simulink model "batteryModel"  (R2024b)
settings: Solver=VariableStepAuto  StartTime=0.0  StopTime=10.0  RelTol=1e-3
model workspace (MAT data in the model file):
  Capacity__Ah_ = 3
  dt = 0.001
undefined symbols (not defined in the file or in its folder): C1_array, Crate_vector, OCV_matrix, R0_array, R1_array, SOC_common, temp_vector
settings Model: Creator=xoxi.1  LastModifiedBy=xoxi.1

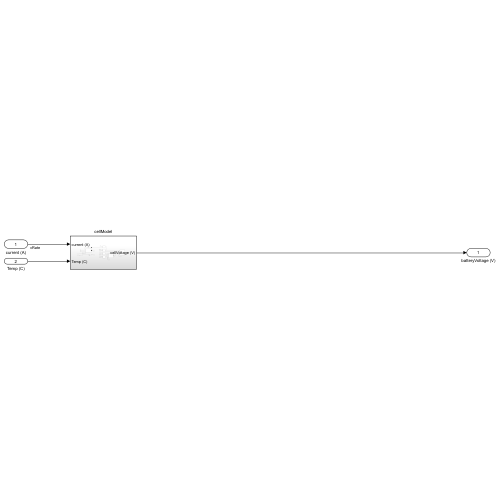
[thumbnail: Simulink's stored preview of the top-level diagram]
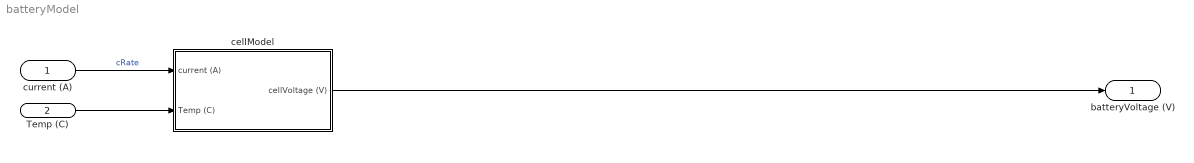
== system batteryModel ==
  current (A) : Inport
  Temp (C) : Inport  Port=2
  cellModel : Subsystem
  batteryVoltage (V) : Outport
  wires:
  current (A)/1 -> cellModel/1(current (A))  "cRate"
  Temp (C)/1 -> cellModel/2(Temp (C))
  cellModel/1(cellVoltage (V)) -> batteryVoltage (V)/1

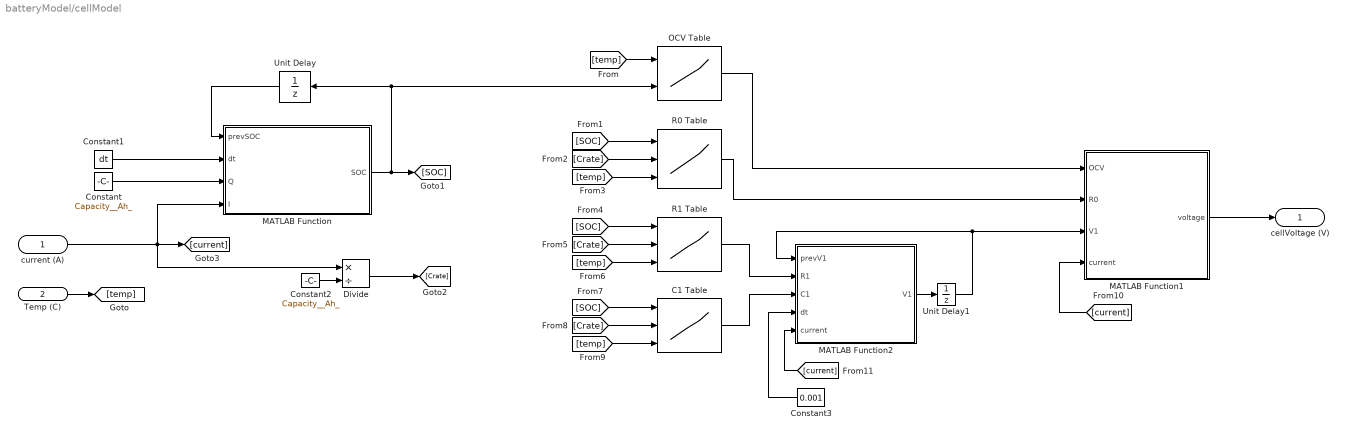
== system batteryModel/cellModel ==
  current (A) : Inport
  Temp (C) : Inport  Port=2
  C1 Table : Lookup_n-D  NumberOfTableDimensions=3  BreakpointsForDimension1=SOC_common  BreakpointsForDimension2=Crate_vector  BreakpointsForDimension3=temp_vector  Table=C1_array  InternalRulePriority=Speed  RndMeth=Simplest
      settings: InputPortMap=u0,u1,u2
  Constant : Constant  Value=Capacity__Ah_
  Constant1 : Constant  Value=dt
  Constant2 : Constant  Value=Capacity__Ah_
  Constant3 : Constant  Value=0.001
  Divide : Product  Inputs=*/
  MATLAB Function : MATLAB Function  TreatAsAtomicUnit=on
  MATLAB Function1 : MATLAB Function  TreatAsAtomicUnit=on
  MATLAB Function2 : MATLAB Function  TreatAsAtomicUnit=on
  OCV Table : Lookup_n-D  BreakpointsForDimension1=temp_vector  BreakpointsForDimension2=SOC_common  Table=OCV_matrix  InternalRulePriority=Speed  RndMeth=Simplest
      settings: InputPortMap=u0,u1
  R0 Table : Lookup_n-D  NumberOfTableDimensions=3  BreakpointsForDimension1=SOC_common  BreakpointsForDimension2=Crate_vector  BreakpointsForDimension3=temp_vector  Table=R0_array  InternalRulePriority=Speed  RndMeth=Simplest
      settings: InputPortMap=u0,u1,u2
  R1 Table : Lookup_n-D  NumberOfTableDimensions=3  BreakpointsForDimension1=SOC_common  BreakpointsForDimension2=Crate_vector  BreakpointsForDimension3=temp_vector  Table=R1_array  InternalRulePriority=Speed  RndMeth=Simplest
      settings: InputPortMap=u0,u1,u2
  Unit Delay : UnitDelay  InitialCondition=1  SampleTime=-1  HasFrameUpgradeWarning=on
  Unit Delay1 : UnitDelay  SampleTime=-1  HasFrameUpgradeWarning=on
  cellVoltage (V) : Outport
  wires:
  R0 Table/1 -> MATLAB Function1/2(R0)
  Unit Delay/1 -> MATLAB Function/1(prevSOC)
  [SOC] -> R0 Table/1
  current (A)/1 -> [current], Divide/1, MATLAB Function/4(I)
  [Crate] -> C1 Table/2
  Constant3/1 -> MATLAB Function2/4(dt)
  Constant1/1 -> MATLAB Function/2(dt)
  [temp] -> C1 Table/3
  [temp] -> R0 Table/3
  [current] -> MATLAB Function2/5(current)
  MATLAB Function1/1(voltage) -> cellVoltage (V)/1
  [temp] -> OCV Table/1
  R1 Table/1 -> MATLAB Function2/2(R1)
  [SOC] -> R1 Table/1
  Constant/1 -> MATLAB Function/3(Q)
  [current] -> MATLAB Function1/4(current)
  Divide/1 -> [Crate]
  Temp (C)/1 -> [temp]
  [SOC] -> C1 Table/1
  MATLAB Function/1(SOC) -> [SOC], Unit Delay/1, OCV Table/2
  MATLAB Function2/1(V1) -> Unit Delay1/1
  [temp] -> R1 Table/3
  Constant2/1 -> Divide/2
  [Crate] -> R0 Table/2
  [Crate] -> R1 Table/2
  OCV Table/1 -> MATLAB Function1/1(OCV)
  Unit Delay1/1 -> MATLAB Function1/3(V1), MATLAB Function2/1(prevV1)
  C1 Table/1 -> MATLAB Function2/3(C1)

== matlab function batteryModel/cellModel/MATLAB Function1 ==
  data: voltage output; OCV input; R0 input; V1 input; current input
function voltage = calculate_voltage(OCV, R0, V1, current)

voltage = OCV - (current * R0) - V1;

end

== matlab function batteryModel/cellModel/MATLAB Function ==
  data: prevSOC input; dt input; Q input; I input; SOC output
function SOC = calculateSOC(prevSOC, dt, Q, I)

SOC = prevSOC - (I * dt) / (Q * 3600);

end

== matlab function batteryModel/cellModel/MATLAB Function2 ==
  data: prevV1 input; R1 input; V1 output; C1 input; dt input; current input
function V1 = calculateV1(prevV1, R1, C1, dt, current)

tao = R1 * C1;

V1 = exp(-dt / tao) * prevV1 + R1 * (1 - exp(-dt / tao)) * current;

end
